simulink model "mass_spring_damper"  (R2024a)
settings: Solver=ode1  StartTime=0.0  StopTime=20  FixedStep=0.1  RelTol=1e-3
undefined symbols (not defined in the file): c, K, k, lambda, m, phi
settings Model: Creator=Lenovo  LastModifiedBy=Lenovo

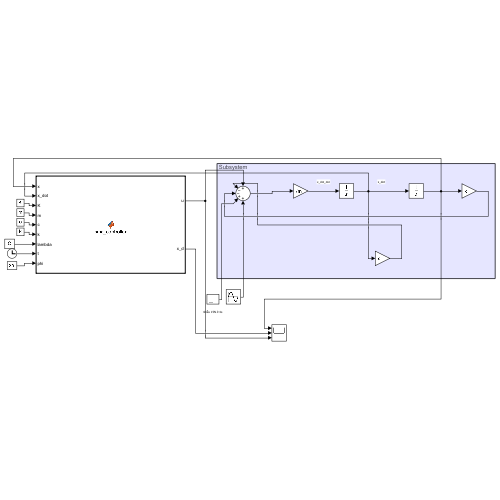
[thumbnail: Simulink's stored preview of the top-level diagram]
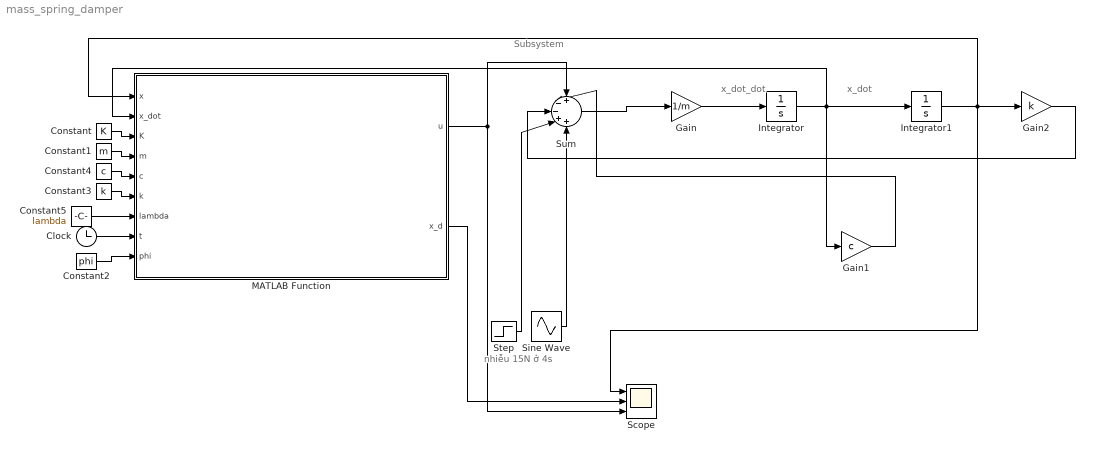
== system mass_spring_damper ==
  note: nhiễu 15N ở 4s
  note: Subsystem
  note: x_dot_dot
  note: x_dot
  Clock : Clock
  Constant : Constant  Value=K
  Constant1 : Constant  Value=m
  Constant2 : Constant  Value=phi
  Constant3 : Constant  Value=k
  Constant4 : Constant  Value=c
  Constant5 : Constant  Value=lambda
  Gain : Gain  Gain=1/m
  Gain1 : Gain  Gain=c
  Gain2 : Gain  Gain=k
  Integrator : Integrator
  Integrator1 : Integrator  InitialCondition=2
  MATLAB Function : MATLAB Function  TreatAsAtomicUnit=on
  Scope : Scope  NumInputPorts=3
  Sine Wave : Sin  Amplitude=10  Frequency=3  SampleTime=0
  Step : Step  Time=4  After=15  SampleTime=0
  Sum : Sum  Inputs=+--++
  wires:
  Integrator1/1 -> Scope/1, MATLAB Function/1(x), Gain2/1
  Gain/1 -> Integrator/1
  Gain1/1 -> Sum/2
  Gain2/1 -> Sum/3
  Sum/1 -> Gain/1
  Integrator/1 -> MATLAB Function/2(x_dot), Gain1/1, Integrator1/1
  Constant/1 -> MATLAB Function/3(K)
  Constant1/1 -> MATLAB Function/4(m)
  MATLAB Function/1(u) -> Sum/1, Scope/3
  Constant3/1 -> MATLAB Function/6(k)
  Constant4/1 -> MATLAB Function/5(c)
  Constant5/1 -> MATLAB Function/7(lambda)
  MATLAB Function/2(x_d) -> Scope/2
  Clock/1 -> MATLAB Function/8(t)
  Constant2/1 -> MATLAB Function/9(phi)
  Sine Wave/1 -> Sum/5
  Step/1 -> Sum/4

== matlab function mass_spring_damper/MATLAB Function ==
  data: x input; u output; x_dot input; K input; m input; c input; k input; lambda input; x_d output; t input; phi input
function [u, x_d] = smc_controller(x, x_dot, K, m, c, k, lambda, t, phi)
x_d = 0;
x_d_dot = 0;
x_d_dot_dot = 0;
e = x - x_d;
e_dot = x_dot - x_d_dot;
s = e_dot + lambda*e;
u_eq = c*x_dot + k*x + m*(x_d_dot_dot - lambda*e_dot);
u_sw = -K*(s/(abs(s)+phi));
u = u_eq + u_sw;
end
